simulink model "test_blocks"  (R2025b)
settings: Solver=VariableStepAuto  StartTime=0.0  StopTime=10.0  RelTol=1e-3
undefined symbols (not defined in the file): SNR, Ts
libraries: commdigbbndpm3 x2, commsink2 x1, dspsrcs4 x1
settings Model: Creator=Пётр  LastModifiedBy=Пётр

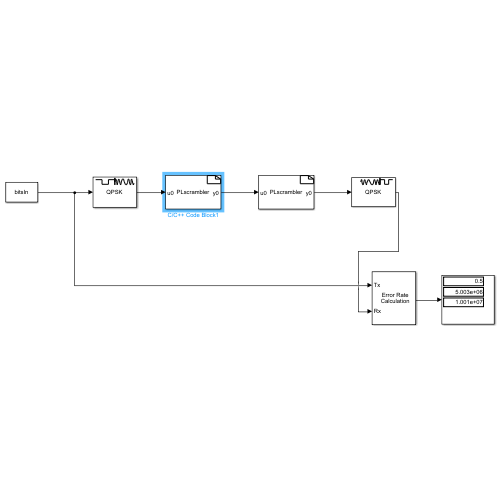
[thumbnail: Simulink's stored preview of the top-level diagram]
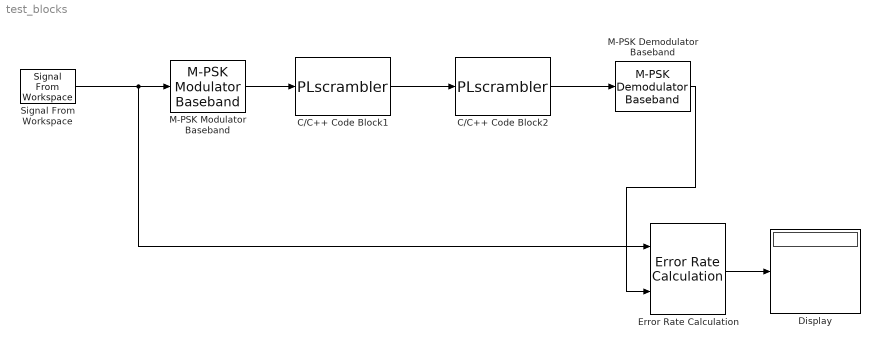
== system test_blocks ==
  C/C++ Code Block1 : S-Function  FunctionName=PLscrambler  SFunctionModules=PLscrambler_wrapper.cpp  SFunctionDeploymentMode=off  EnableBusSupport=off  mask(S-Function Builder){}
      mask help: Simulink:masks:SFunctionBuilder_MD
      mask init:
      | val = [[.9  0.75 0.75 1 1 .9 .9 1]',[1 1 0.75 0.75 .9 .9 1 .9]'];try , sys = get_param(gcb,'SfunBuilderFcnName');if isempty(sys), sys = get_param(gcb,'FunctionName'); end,catch, sys = get_param(gcb,'FunctionName'); end
      settings: CopyFcn=set_param(gcbh,'LinkStatus','none')  OpenFcn=sfunctionwizard(gcbh)
      mask Display:
      | plot(val(:,1),val(:,2))
      | disp(sys)
      | port_label('input',1,sprintf('%s', 'u0'),'interpreter','tex')
      | port_label('output',1,sprintf('%s', 'y0'),'interpreter','tex')
  C/C++ Code Block2 : S-Function  FunctionName=PLscrambler  SFunctionModules=PLscrambler_wrapper.cpp  SFunctionDeploymentMode=off  EnableBusSupport=off  mask(S-Function Builder){}
      mask help: Simulink:masks:SFunctionBuilder_MD
      mask init: same as test_blocks/C/C++ Code Block1
      settings: CopyFcn=set_param(gcbh,'LinkStatus','none')  OpenFcn=sfunctionwizard(gcbh)
      mask Display:
      | plot(val(:,1),val(:,2))
      | disp(sys)
      | port_label('input',1,sprintf('%s', 'u0'),'interpreter','tex')
      | port_label('output',1,sprintf('%s', 'y0'),'interpreter','tex')
  Display : Display
  Error Rate Calculation : commsink2/Error Rate Calculation  N=6312  st_delay=0  cp_mode=Entire frame  subframe=[]  PMode=Port  WsName=ErrorVec  RsMode2=off  stop=off  numErr=100  maxBits=1e6
  M-PSK Demodulator Baseband : commdigbbndpm3/M-PSK Demodulator Baseband  M=4  OutType=Bit  DecType=Hard decision  VarSource=Dialog  Variance=1 / (2 * 10^(SNR/10))  Dec=User-defined  Mapping=[0 2 3 1]  Ph=pi/4  outDtype1=boolean  outDtype2=Inherit via internal rule  derotateFactorWordLen=16  derotateFactorDataTypeStr=Inherit: Same word length as input  derotateFactorLastDataTypeStr=Inherit: Same word length as input
  M-PSK Modulator Baseband : commdigbbndpm3/M-PSK Modulator Baseband  M=4  InType=Bit  Enc=User-defined  Mapping=[0 2 3 1]  Ph=pi/4  outDtype=double  outWordLen=16  outUDDataType=sfix(16)  outFracLenMode=Best precision  outFracLen=15  outDataTypeStr=double  outLastDataTypeStr=double
  Signal From Workspace : dspsrcs4/Signal From Workspace  X=bitsIn  Ts=Ts  nsamps=16200  OutputAfterFinalValue=Setting to zero  ignoreOrWarnInputAndFrameLengths=off  OutputFrames=off
  wires:
  C/C++ Code Block1/1 -> C/C++ Code Block2/1
  M-PSK Modulator Baseband/1 -> C/C++ Code Block1/1
  C/C++ Code Block2/1 -> M-PSK Demodulator Baseband/1
  Error Rate Calculation/1 -> Display/1
  Signal From Workspace/1 -> Error Rate Calculation/1, M-PSK Modulator Baseband/1
  M-PSK Demodulator Baseband/1 -> Error Rate Calculation/2
